simulink subsystem "ALU"  (R2024b)
settings: Solver=VariableStepAuto  StartTime=0.0  StopTime=10.0  RelTol=1e-3
libraries: hdlsllib x9, simulink x5
settings Model: Creator=stefano  LastModifiedBy=stefano
settings RTWCC: GPUComputeCapability=3.5

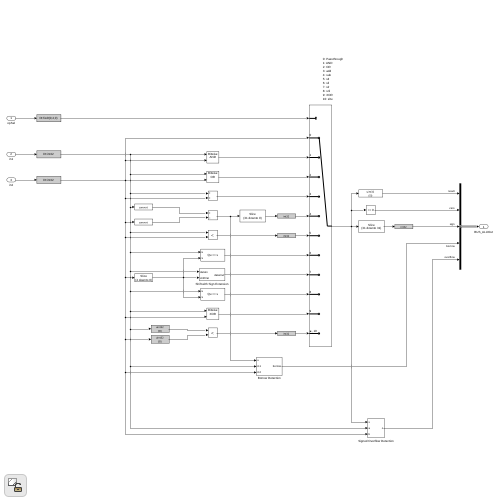
[thumbnail: Simulink's stored preview of the top-level diagram]
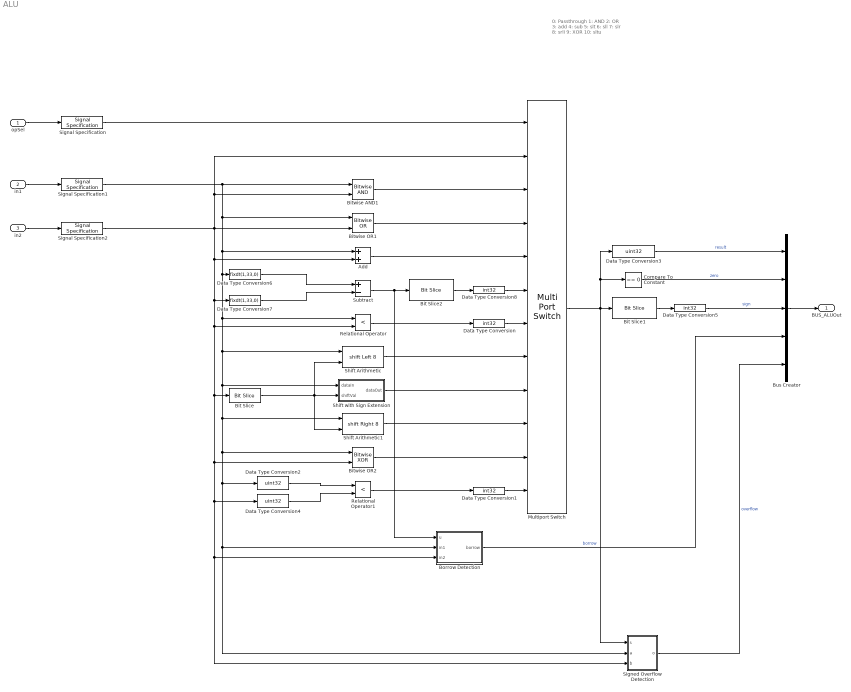
== system ALU ==
  note: 0: Passthrough
      | 1: AND
      | 2: OR
      | 3: add
      | 4: sub
      | 5: slt
      | 6: sll
      | 7: slr
      | 8: srli
      | 9: XOR
      | 10: sltu
  opSel : Inport
  in1 : Inport  Port=2
  in2 : Inport  Port=3
  Add : Sum
  Bit Slice : hdlsllib/Logic and Bit Operations/Bit Slice  lidx=4  ridx=0
  Bit Slice1 : hdlsllib/Logic and Bit Operations/Bit Slice  lidx=31  ridx=31
  Bit Slice2 : hdlsllib/Logic and Bit Operations/Bit Slice  lidx=31  ridx=0
  Bitwise AND1 : simulink/Logic and Bit Operations/Bitwise Operator  logicop=AND  UseBitMask=off  NumInputPorts=2  BitMask=bin2dec('11011001')  BitMaskRealWorld=Stored Integer
      settings: LibrarySourceBlock=|
      | simulink/Quick Insert/Logic and Bit
      | Operations/Bitwise AND
  Bitwise OR1 : simulink/Logic and Bit Operations/Bitwise Operator  logicop=OR  UseBitMask=off  NumInputPorts=2  BitMask=bin2dec('11011001')  BitMaskRealWorld=Stored Integer
      settings: LibrarySourceBlock=|
      | simulink/Quick Insert/Logic and Bit
      | Operations/Bitwise OR
  Bitwise OR2 : simulink/Logic and Bit Operations/Bitwise Operator  logicop=XOR  UseBitMask=off  NumInputPorts=2  BitMask=bin2dec('11011001')  BitMaskRealWorld=Stored Integer
      settings: LibrarySourceBlock=|
      | simulink/Quick Insert/Logic and Bit
      | Operations/Bitwise OR
  Borrow Detection : Subsystem
  Bus Creator : BusCreator  Inputs=5
  Compare To Constant : simulink/Logic and Bit Operations/Compare To Constant  relop===  const=0  OutDataTypeStr=boolean
  Data Type Conversion{,1,5,8} (4 alike) : DataTypeConversion  OutDataTypeStr=int32  SaturateOnIntegerOverflow=off  RndMeth=Floor
  Data Type Conversion2 : DataTypeConversion  OutDataTypeStr=uint32  ConvertRealWorld=Stored Integer (SI)  SaturateOnIntegerOverflow=off  RndMeth=Floor
  Data Type Conversion3 : DataTypeConversion  OutDataTypeStr=uint32  ConvertRealWorld=Stored Integer (SI)  SaturateOnIntegerOverflow=off  RndMeth=Floor
  Data Type Conversion4 : DataTypeConversion  OutDataTypeStr=uint32  ConvertRealWorld=Stored Integer (SI)  SaturateOnIntegerOverflow=off  RndMeth=Floor
  Data Type Conversion6 : DataTypeConversion  OutDataTypeStr=fixdt(1,33,0)  SaturateOnIntegerOverflow=off  RndMeth=Floor
  Data Type Conversion7 : DataTypeConversion  OutDataTypeStr=fixdt(1,33,0)  SaturateOnIntegerOverflow=off  RndMeth=Floor
  Multiport Switch : MultiPortSwitch  DataPortOrder=Zero-based contiguous  Inputs=11  DiagnosticForDefault=Warning  zeroidx=on  SaturateOnIntegerOverflow=off  InputSameDT=off
  Relational Operator : RelationalOperator  Operator=<  OutDataTypeStr=boolean  RndMeth=Simplest  InputSameDT=off
  Relational Operator1 : RelationalOperator  Operator=<  OutDataTypeStr=boolean  RndMeth=Simplest  InputSameDT=off
  Shift Arithmetic : ArithShift  BitShiftNumberSource=Input port  BitShiftNumber=8  BitShiftDirection=Left
      settings: InputPortMap=u0,p1
  Shift Arithmetic1 : ArithShift  BitShiftNumberSource=Input port  BitShiftNumber=8  BitShiftDirection=Right
      settings: InputPortMap=u0,p1
  Shift with Sign Extension : Subsystem
  Signal Specification : SignalSpecification  OutDataTypeStr=fixdt(0,4,0)
  Signal Specification1 : SignalSpecification  OutDataTypeStr=int32
  Signal Specification2 : SignalSpecification  OutDataTypeStr=int32
  Signed Overflow Detection : Subsystem
  Subtract : Sum  Inputs=+-  OutDataTypeStr=Inherit: Same as first input
  BUS_ALUOut : Outport
  wires:
  Borrow Detection/1(borrow) -> Bus Creator/4  "borrow"
  Bus Creator/1 -> BUS_ALUOut/1
  Signed Overflow Detection/1(o) -> Bus Creator/5  "overflow"
  Signal Specification1/1 -> Bitwise AND1/1, Bitwise OR1/1, Add/1, Relational Operator/1, Borrow Detection/2(in1), Signed Overflow Detection/2(a), Data Type Conversion2/1, Bitwise OR2/1, Shift Arithmetic1/1, Shift with Sign Extension/1(dataIn), Shift Arithmetic/1, Data Type Conversion6/1
  Data Type Conversion5/1 -> Bus Creator/3  "sign"
  Bit Slice1/1 -> Data Type Conversion5/1
  Data Type Conversion4/1 -> Relational Operator1/2
  Data Type Conversion2/1 -> Relational Operator1/1
  Data Type Conversion1/1 -> Multiport Switch/12
  Relational Operator1/1 -> Data Type Conversion1/1
  Signal Specification2/1 -> Bitwise OR1/2, Add/2, Data Type Conversion7/1, Signed Overflow Detection/3(b), Borrow Detection/3(in2), Data Type Conversion4/1, Bitwise OR2/2, Bit Slice/1, Relational Operator/2, Multiport Switch/2, Bitwise AND1/2
  Bitwise OR2/1 -> Multiport Switch/11
  Shift Arithmetic1/1 -> Multiport Switch/10
  Shift with Sign Extension/1(dataOut) -> Multiport Switch/9
  Bit Slice/1 -> Shift Arithmetic1/2, Shift Arithmetic/2, Shift with Sign Extension/2(shiftVal)
  Shift Arithmetic/1 -> Multiport Switch/8
  Data Type Conversion3/1 -> Bus Creator/1  "result"
  Data Type Conversion/1 -> Multiport Switch/7
  Relational Operator/1 -> Data Type Conversion/1
  Subtract/1 -> Borrow Detection/1(u), Bit Slice2/1
  Add/1 -> Multiport Switch/5
  Bitwise OR1/1 -> Multiport Switch/4
  Bitwise AND1/1 -> Multiport Switch/3
  Signal Specification/1 -> Multiport Switch/1
  Multiport Switch/1 -> Data Type Conversion3/1, Compare To Constant/1, Bit Slice1/1, Signed Overflow Detection/1(s)
  in2/1 -> Signal Specification2/1
  in1/1 -> Signal Specification1/1
  opSel/1 -> Signal Specification/1
  Compare To Constant/1 -> Bus Creator/2  "zero"
  Data Type Conversion6/1 -> Subtract/1
  Data Type Conversion7/1 -> Subtract/2
  Bit Slice2/1 -> Data Type Conversion8/1
  Data Type Conversion8/1 -> Multiport Switch/6

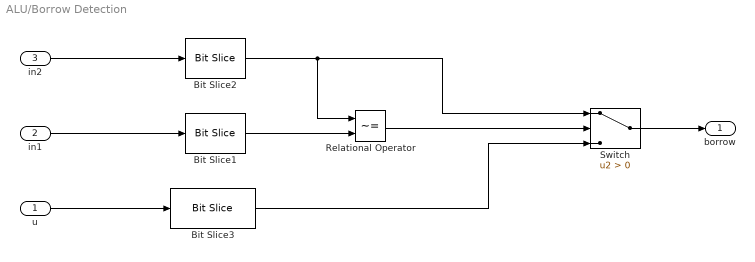
== system ALU/Borrow Detection ==
  u : Inport
  in1 : Inport  Port=2
  in2 : Inport  Port=3
  Bit Slice1 : hdlsllib/Logic and Bit Operations/Bit Slice  lidx=31  ridx=31
  Bit Slice2 : hdlsllib/Logic and Bit Operations/Bit Slice  lidx=31  ridx=31
  Bit Slice3 : hdlsllib/Logic and Bit Operations/Bit Slice  lidx=32  ridx=32
  Relational Operator : RelationalOperator  Operator=~=  OutDataTypeStr=boolean  RndMeth=Simplest  InputSameDT=off
  Switch : Switch  Criteria=u2 > Threshold  SaturateOnIntegerOverflow=off  InputSameDT=off
  borrow : Outport
  wires:
  u/1 -> Bit Slice3/1
  in1/1 -> Bit Slice1/1
  Bit Slice2/1 -> Relational Operator/1, Switch/1
  Bit Slice3/1 -> Switch/3
  Relational Operator/1 -> Switch/2
  in2/1 -> Bit Slice2/1
  Bit Slice1/1 -> Relational Operator/2
  Switch/1 -> borrow/1

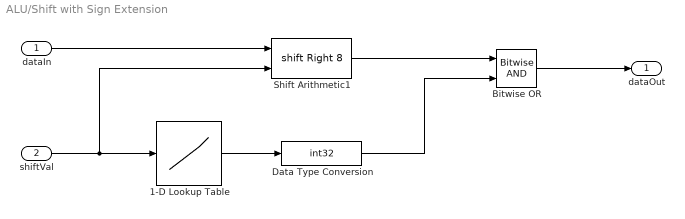
== system ALU/Shift with Sign Extension ==
  dataIn : Inport
  shiftVal : Inport  Port=2
  1-D Lookup Table : Lookup_n-D  NumberOfTableDimensions=1  BreakpointsForDimension1=[0:31]  IndexSearchMethod=Evenly spaced points  Table=(2.^(32:-1:1)-1)  ExtrapMethod=Clip  UseLastTableValue=on  InternalRulePriority=Speed  OutDataTypeStr=uint32  RndMeth=Simplest
  Bitwise OR : simulink/Logic and Bit Operations/Bitwise Operator  logicop=AND  UseBitMask=off  NumInputPorts=2  BitMask=bin2dec('11011001')  BitMaskRealWorld=Stored Integer
  Data Type Conversion : DataTypeConversion  OutDataTypeStr=int32  ConvertRealWorld=Stored Integer (SI)  SaturateOnIntegerOverflow=off  RndMeth=Floor
  Shift Arithmetic1 : ArithShift  BitShiftNumberSource=Input port  BitShiftNumber=8  BitShiftDirection=Right
      settings: InputPortMap=u0,p1
  dataOut : Outport
  wires:
  1-D Lookup Table/1 -> Data Type Conversion/1
  dataIn/1 -> Shift Arithmetic1/1
  Shift Arithmetic1/1 -> Bitwise OR/1
  shiftVal/1 -> 1-D Lookup Table/1, Shift Arithmetic1/2
  Bitwise OR/1 -> dataOut/1
  Data Type Conversion/1 -> Bitwise OR/2

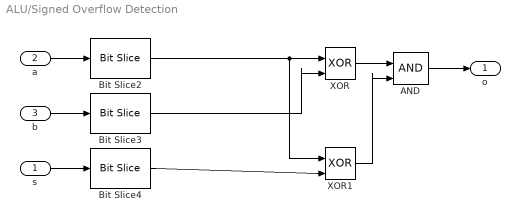
== system ALU/Signed Overflow Detection ==
  s : Inport
  a : Inport  Port=2
  b : Inport  Port=3
  AND : Logic  IconShape=distinctive  AllPortsSameDT=off  OutDataTypeStr=boolean
  Bit Slice2 : hdlsllib/Logic and Bit Operations/Bit Slice  lidx=31  ridx=31
  Bit Slice3 : hdlsllib/Logic and Bit Operations/Bit Slice  lidx=31  ridx=31
  Bit Slice4 : hdlsllib/Logic and Bit Operations/Bit Slice  lidx=31  ridx=31
  XOR : Logic  Operator=XOR  IconShape=distinctive  AllPortsSameDT=off  OutDataTypeStr=boolean
  XOR1 : Logic  Operator=XOR  IconShape=distinctive  AllPortsSameDT=off  OutDataTypeStr=boolean
  o : Outport
  wires:
  AND/1 -> o/1
  Bit Slice4/1 -> XOR1/2
  Bit Slice2/1 -> XOR1/1, XOR/1
  XOR1/1 -> AND/2
  Bit Slice3/1 -> XOR/2
  s/1 -> Bit Slice4/1
  XOR/1 -> AND/1
  b/1 -> Bit Slice3/1
  a/1 -> Bit Slice2/1
